simulink model "EV_TCL"  (R2020a)
settings: Solver=VariableStepAuto  StartTime=0.0  StopTime=2  RelTol=1e-3
values from neighbouring files (symbols this model uses):
  d = 0.2    [Parameters.mat]
  imax = 180    [Parameters.mat]
  Ki = 100    [Parameters.mat]
  Kp = 2.5    [Parameters.mat]
  tol = 1.0e-10    (= 1e-10)    [Prarams_TCL_test.m]
  Tsc = 5e-05    [Parameters.mat]
libraries: ee_lib x14, fl_lib x12, nesl_utility x12, sdl_lib x6, eeDiscretePi x1, eeSrmCurrentController x1
settings Model: Creator=NIKHIL  LastModifiedBy=NIKHIL

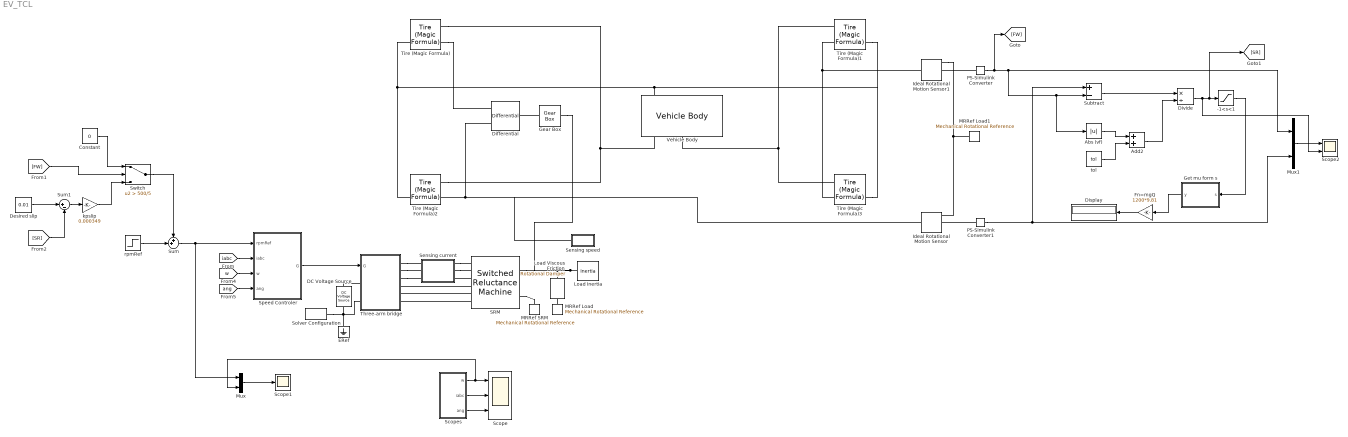
== system EV_TCL ==
  " Speed Controler " : Subsystem
  -1<s<1 : Saturate  UpperLimit=1  LowerLimit=-1
  Abs (vf) : Abs
  Add2 : Sum
  Constant : Constant  Value=0
  DC Voltage Source : fl_lib/Electrical/Electrical Sources/DC Voltage Source  v0=Vdc V
  Desired slip : Constant  Value=0.01
  Differential : sdl_lib/Gears/Differential  driveshaft_location=sdl.enum.differential_orientation.right  cd_ratio=4  friction_model=sdl.enum.gear_friction.none  mu_visc=[0, 0] N*m/(rad/s)  efficiency=[.85, .92]  temperature_TLU=[280, 300, 320] K  efficiency_ss_TLU=[.95, .9, .85]  efficiency_cd_TLU=[.95, .9, .85]  pwr_thr=[.001, .001] W  thermal_mass=50 J/K  T_init=300 K  model_inertia=simscape.enum.onoff.off  carrier_inertia=0.001 kg*m^2  planet_inertia=0.001 kg*m^2
      settings: SourceProductBaseCode=LD
  Display : Display
  Divide : Product  Inputs=*/
  ERef : fl_lib/Electrical/Electrical Elements/Electrical Reference
  Fn=mgQ : Gain  Gain=1200*9.81
  Gear Box : fl_lib/Mechanical/Mechanisms/Gear Box  ratio=5  t_in_specify=off  t_in_priority=None  t_in=0 N*m  t_in_nominal_specify=off  t_in_nominal_unit=N*m  t_in_nominal_value=1  t_out_specify=off  t_out_priority=None  t_out=0 N*m  t_out_nominal_specify=off  t_out_nominal_unit=N*m  t_out_nominal_value=1
  Get mu form s : MATLAB Function  TreatAsAtomicUnit=on
  Ideal Rotational Motion Sensor : fl_lib/Mechanical/Mechanical Sensors/Ideal Rotational Motion Sensor  wrap_angle=simscape.enum.onoff.off  offset=0 rad
  Ideal Rotational Motion Sensor1 : fl_lib/Mechanical/Mechanical Sensors/Ideal Rotational Motion Sensor  wrap_angle=simscape.enum.onoff.off  offset=0 rad
  Load Inertia : fl_lib/Mechanical/Rotational Elements/Inertia  inertia=Jm kg*m^2  w_specify=off  w_priority=High  w=0 rad/s  w_nominal_specify=off  w_nominal_unit=rad/s  w_nominal_value=1  t_specify=off  t_priority=High  t=0 N*m  t_nominal_specify=off  t_nominal_unit=N*m  t_nominal_value=1
  Load Viscous Friction : fl_lib/Mechanical/Rotational Elements/Rotational Damper  D=d N*m/(rad/s)  w_specify=off  w_priority=High  w=0 rad/s  w_nominal_specify=off  w_nominal_unit=rad/s  w_nominal_value=1  t_specify=off  t_priority=High  t=0 N*m  t_nominal_specify=off  t_nominal_unit=N*m  t_nominal_value=1
  MRRef Load : fl_lib/Mechanical/Rotational Elements/Mechanical Rotational Reference
  MRRef Load1 : fl_lib/Mechanical/Rotational Elements/Mechanical Rotational Reference
  MRRef SRM : fl_lib/Mechanical/Rotational Elements/Mechanical Rotational Reference
  Mux : Mux  Inputs=2
  Mux1 : Mux  Inputs=2
  PS-Simulink Converter : nesl_utility/PS-Simulink Converter  PhysicalDomain=network_engine_domain  SubClassName=ps_output  LeftPortType=input  RightPortType=output  PseudoPeriodic=off  Frequencies=[]  Unit=inherit  AffineConversion=off
  PS-Simulink Converter1 : nesl_utility/PS-Simulink Converter  PhysicalDomain=network_engine_domain  SubClassName=ps_output  LeftPortType=input  RightPortType=output  PseudoPeriodic=off  Frequencies=[]  Unit=inherit  AffineConversion=off
  SRM : ee_lib/Electromechanical/Reluctance & Stepper/Switched Reluctance Machine  nPoleRotor=p  Rs=Rs Ohm  stator_param=3  Rm=inf Ohm  psi_sat=0.43 Wb  Lmax=0.0046 H  Lmin=6.7e-4 H  thetaS=45 deg  thetaR=42 deg  thetaSmoothing=0.5 deg  J=0 kg*m^2  lam=0 N*m/(rad/s)  iVec=iph A  xVec=th rad  FluxMatrix=psi Wb  i_a_specify=off  i_a_priority=None  i_a=0 A  i_a_nominal_specify=off  i_a_nominal_unit=A  i_a_nominal_value=1  i_b_specify=off  i_b_priority=None  i_b=0 A  i_b_nominal_specify=off  i_b_nominal_unit=A  i_b_nominal_value=1  i_c_specify=off  i_c_priority=None  i_c=0 A  i_c_nominal_specify=off  i_c_nominal_unit=A  i_c_nominal_value=1  torque_specify=off  torque_priority=None  torque=0 N*m  torque_nominal_specify=off  torque_nominal_unit=N*m  torque_nominal_value=1  angular_velocity_specify=off  angular_velocity_priority=High  angular_velocity=0 rpm  angular_velocity_nominal_specify=off  angular_velocity_nominal_unit=rpm  angular_velocity_nominal_value=1  angular_position_diff_specify=on  angular_position_diff_priority=High  angular_position_diff=0 deg  angular_position_diff_nominal_specify=off  angular_position_diff_nominal_unit=deg  angular_position_diff_nominal_value=1  alpha=3.93e-3 1/K  Tmeas=25 degC  thermal_mass=100 J/K  rotor_thermal_mass=50 J/K  Rm_percent_rotor=50  temperatureA_specify=off  temperatureA_priority=High  temperatureA=25 degC  temperatureA_nominal_specify=off  temperatureA_nominal_unit=degC  temperatureA_nominal_value=1  temperatureB_specify=off  temperatureB_priority=High  temperatureB=25 degC  temperatureB_nominal_specify=off  temperatureB_nominal_unit=degC  temperatureB_nominal_value=1  temperatureC_specify=off  temperatureC_priority=High  temperatureC=25 degC  temperatureC_nominal_specify=off  temperatureC_nominal_unit=degC  temperatureC_nominal_value=1  temperatureR_specify=off  temperatureR_priority=High  temperatureR=25 degC  temperatureR_nominal_specify=off  temperatureR_nominal_unit=degC  temperatureR_nominal_value=1
      settings: SourceProductBaseCode=PS  InternalSimscapePortConfiguration="{\"Bottom\":[],\"Left\":[{\"id\":\"a1\",\"label\":\"a1\",\"type\":\"foundation.electrical.electrical\"},{\"id\":\"b1\",\"label\":\"b1\",\"type\":\"foundation.electrical.electrical\"},{\"id\":\"c1\",\"label\":\"c1\",\"type\":\"foundation.electrical.electrical\"},{\"id\":\"a2\",\"label\":\"a2\",\"type\":\"foundation.electrical.electrical\"},{\"id\":\"b2\",\"label\":\"b2\",\"type\":\"foundation.electrical.electrical\"},{\"id\":\"c2\",\"label\":\"c2\",\"type\":\"foundation.electrical.electrical\"}],\"Right\":[{\"id\":\"R\",\"label\":\"R\",\"type\":\"foundation.mechanical.rotational.rotational\"},{\"id\":\"C\",\"label\":\"C\",\"type\":\"foundation.mechanical.rotational.rotational\"}],\"Top\":[]}"
  Scope : Scope  NumInputPorts=3
  Scope1 : Scope
  Scope2 : Scope  NumInputPorts=2
  Scopes : Subsystem
  Sensing current : Subsystem
      mask Display: disp('iabc')
  Sensing speed : Subsystem
      mask Display: disp('w,ang')
  Solver Configuration : nesl_utility/Solver Configuration  PhysicalDomain=network_engine_domain  SubClassName=solver  LeftPortType=input  RightPortType=generic  Tones=[]  Harmonics=[]  SimulateNoise=off  Profile=off  UseLocalSampling=off  EnableSwitchedLinearOptims=on  FrequencyDomain=off  UseCCode=off  RelTol=0.001  AbsTol=1e-06  MinStep=1e-09  ToWorkspace=off  RevertToSquareIcSolve=off  NumHomotopyIterations=100  PhasorMode=off  PhasorModeNumHarmonics=1  DoDC=off  ResidualTolerance=1e-9  UseLocalSolver=on  LocalSolverChoice=NE_BACKWARD_EULER_ADVANCER  LocalSolverSampleTime=Ts  DoFixedCost=on  MaxNonlinIter=5  MaxModeIter=2  LinearAlgebra=auto  EquationFormulation=NE_TIME_EF  DelaysMemoryBudget=1024  AutomaticFiltering=on  FilteringTimeConstant=0.001  PartitionStorageMethod=AS_NEEDED  PartitionMemoryBudget=1024  PartitionMethod=FAST
  Subtract : Sum  Inputs=+-
  Sum : Sum  Inputs=++|
  Sum1 : Sum  Inputs=|+-
  Switch : Switch  Criteria=u2 > Threshold  Threshold=500/5
  Three-arm bridge : Subsystem  Tag=PublishSubsystem
  Tire (Magic Formula) : sdl_lib/Tires & Vehicles/Tire (Magic Formula)  parameterization=sdl.enum.magic_tire_model.peak  F_z1=3000 N  F_x1=3500 N  kappa1=20  B_m=10  C_m=1.9  D_m=1  E_m=0.97  fz0=4000 N  p_Cx=1.685  p_Dx=[1.21, -.037]  p_Ex=[.344, .095, -.02, 0]  p_Kx=[21.51, -.163, .245]  p_Hx=[-.002, .002]  p_Vx=[0, 0]  v_tr_thr=0.1 m/s  r_e=0.3 m  model_compliance=0  stiffness=1e6 N/m  damping=1000 N/(m/s)  model_inertia=0  inertia=1 kg*m^2  initial_velocity=0 rad/s  model_resistance=0  resistance_model=1  coeff=0.015  p_tire=250e3 Pa  alpha=-0.003  beta=0.97  coeff_a=84e-4  coeff_b=6.2e-4 s/m  coeff_c=1.6e-4 s^2/m^2  v_thr=0.001 m/s
  Tire (Magic Formula)1 : sdl_lib/Tires & Vehicles/Tire (Magic Formula)  parameterization=sdl.enum.magic_tire_model.peak  F_z1=3000 N  F_x1=3500 N  kappa1=10  B_m=10  C_m=1.9  D_m=1  E_m=0.97  fz0=4000 N  p_Cx=1.685  p_Dx=[1.21, -.037]  p_Ex=[.344, .095, -.02, 0]  p_Kx=[21.51, -.163, .245]  p_Hx=[-.002, .002]  p_Vx=[0, 0]  v_tr_thr=0.1 m/s  r_e=0.3 m  model_compliance=0  stiffness=1e6 N/m  damping=1000 N/(m/s)  model_inertia=0  inertia=1 kg*m^2  initial_velocity=0 rad/s  model_resistance=0  resistance_model=1  coeff=0.015  p_tire=250e3 Pa  alpha=-0.003  beta=0.97  coeff_a=84e-4  coeff_b=6.2e-4 s/m  coeff_c=1.6e-4 s^2/m^2  v_thr=0.001 m/s
  Tire (Magic Formula)2 : sdl_lib/Tires & Vehicles/Tire (Magic Formula)  parameterization=sdl.enum.magic_tire_model.peak  F_z1=3000 N  F_x1=3500 N  kappa1=20  B_m=10  C_m=1.9  D_m=1  E_m=0.97  fz0=4000 N  p_Cx=1.685  p_Dx=[1.21, -.037]  p_Ex=[.344, .095, -.02, 0]  p_Kx=[21.51, -.163, .245]  p_Hx=[-.002, .002]  p_Vx=[0, 0]  v_tr_thr=0.1 m/s  r_e=0.3 m  model_compliance=0  stiffness=1e6 N/m  damping=1000 N/(m/s)  model_inertia=0  inertia=1 kg*m^2  initial_velocity=0 rad/s  model_resistance=0  resistance_model=1  coeff=0.015  p_tire=250e3 Pa  alpha=-0.003  beta=0.97  coeff_a=84e-4  coeff_b=6.2e-4 s/m  coeff_c=1.6e-4 s^2/m^2  v_thr=0.001 m/s
  Tire (Magic Formula)3 : sdl_lib/Tires & Vehicles/Tire (Magic Formula)  parameterization=sdl.enum.magic_tire_model.peak  F_z1=3000 N  F_x1=3500 N  kappa1=10  B_m=10  C_m=1.9  D_m=1  E_m=0.97  fz0=4000 N  p_Cx=1.685  p_Dx=[1.21, -.037]  p_Ex=[.344, .095, -.02, 0]  p_Kx=[21.51, -.163, .245]  p_Hx=[-.002, .002]  p_Vx=[0, 0]  v_tr_thr=0.1 m/s  r_e=0.3 m  model_compliance=0  stiffness=1e6 N/m  damping=1000 N/(m/s)  model_inertia=0  inertia=1 kg*m^2  initial_velocity=0 rad/s  model_resistance=0  resistance_model=1  coeff=0.015  p_tire=250e3 Pa  alpha=-0.003  beta=0.97  coeff_a=84e-4  coeff_b=6.2e-4 s/m  coeff_c=1.6e-4 s^2/m^2  v_thr=0.001 m/s
  Vehicle Body : sdl_lib/Tires & Vehicles/Vehicle Body  mass=1200 kg  n_w=2  x_f=1.4 m  x_r=1.6 m  y_c=0.5 m  mass_var=simscape.enum.onoff.off  model_pitch=simscape.enum.onoff.off  inertia=4000 kg*m^2  suspension_model=sdl.enum.linearTLU.linear  k_f=1e4 N/m  b_f=1e4 N/(m/s)  k_r=1e4 N/m  b_r=1e4 N/(m/s)  k_f_TLU=[-2000, -1000, 0, 1000, 2000] N  x_f_TLU=[-.4, -.2, 0, .2, .4] m  b_f_TLU=[-200, -100, 0, 100, 200] N  v_f_TLU=[-4, -2, 0, 2, 4] m/s  k_r_TLU=[-2000, -1000, 0, 1000, 2000] N  x_r_TLU=[-.4, -.2, 0, .2, .4] m  b_r_TLU=[-200, -100, 0, 100, 200] N  v_r_TLU=[-4, -2, 0, 2, 4] m/s  interp_method=simscape.enum.interpolation.linear  extrap_method=simscape.enum.extrapolation.linear  model_hardstop=simscape.enum.onoff.off  upper_bound_f=.25 m  lower_bound_f=-.25 m  stop_k_f=1e6 N/m  stop_b_f=150 N/(m/s)  upper_bound_r=.25 m  lower_bound_r=-.25 m  stop_k_r=1e6 N/m  stop_b_r=150 N/(m/s)  initial_pitch=0 rad  initial_pitch_rate=0 rad/s  g=9.81 m/s^2  liftoff_warning=simscape.enum.onoff.off  area=3 m^2  Cd=0.4  rho=1.18 kg/m^3  v_specify=off  v_priority=High  v=0 m/s  v_nominal_specify=off  v_nominal_unit=m/s  v_nominal_value=1
  kpslip : Gain  Gain=0.000349
  rpmRef : Step  Time=0.5  After=500  SampleTime=0
  tol : Constant  Value=tol
  wires:
  Mux/1 -> Scope1/1
  [iabc] -> " Speed Controler "/2(iabc)
  Scopes/2(iabc) -> Scope/2
  Scopes/3(ang) -> Scope/3
  Scopes/1(w) -> Mux/2, Scope/1
  " Speed Controler "/1(G) -> Three-arm bridge/1(G)
  [w] -> " Speed Controler "/3(w)
  [ang] -> " Speed Controler "/4(ang)
  Mux1/1 -> Scope2/1
  -1<s<1/1 -> Get mu form s/1(s)
  tol/1 -> Add2/2
  Divide/1 -> Scope2/2, [SR], -1<s<1/1
  Add2/1 -> Divide/2
  Get mu form s/1(y) -> Fn=mgQ/1
  Fn=mgQ/1 -> Display/1
  Abs (vf)/1 -> Add2/1
  Subtract/1 -> Divide/1
  PS-Simulink Converter1/1 -> Mux1/2, Subtract/1
  PS-Simulink Converter/1 -> [FW], Abs (vf)/1, Subtract/2, Mux1/1
  Constant/1 -> Switch/1
  Sum1/1 -> kpslip/1
  Desired slip/1 -> Sum1/1
  kpslip/1 -> Switch/3
  [FW] -> Switch/2
  [SR] -> Sum1/2
  rpmRef/1 -> Sum/2
  Sum/1 -> Mux/1, " Speed Controler "/1(rpmRef)
  Switch/1 -> Sum/1
  connections:
  Differential/RConn2 -- Sensing speed/LConn1 -- Ideal Rotational Motion Sensor/LConn1 -- Tire (Magic Formula)2/LConn2
  Tire (Magic Formula)/LConn2 -- Differential/RConn1
  Gear Box/LConn1 -- Differential/LConn1
  Vehicle Body/LConn1 -- Tire (Magic Formula)1/RConn2 -- Tire (Magic Formula)3/RConn2 -- Tire (Magic Formula)2/RConn2 -- Tire (Magic Formula)/RConn2
  Tire (Magic Formula)/LConn1 -- Tire (Magic Formula)2/LConn1 -- Vehicle Body/RConn1
  Tire (Magic Formula)1/LConn1 -- Tire (Magic Formula)3/LConn1 -- Vehicle Body/RConn2
  Tire (Magic Formula)3/LConn2 -- Ideal Rotational Motion Sensor1/LConn1 -- Tire (Magic Formula)1/LConn2
  Solver Configuration/RConn1 -- ERef/LConn1 -- DC Voltage Source/RConn1 -- Three-arm bridge/LConn2
  Load Inertia/LConn1 -- Gear Box/RConn1 -- SRM/RConn1 -- Load Viscous Friction/LConn1
  SRM/LConn5 -- Three-arm bridge/RConn5
  Sensing current/RConn1 -- SRM/LConn1
  SRM/LConn4 -- Three-arm bridge/RConn4
  Three-arm bridge/LConn1 -- DC Voltage Source/LConn1
  SRM/LConn6 -- Three-arm bridge/RConn6
  SRM/RConn2 -- MRRef SRM/LConn1
  Three-arm bridge/RConn3 -- Sensing current/LConn3
  Three-arm bridge/RConn2 -- Sensing current/LConn2
  Three-arm bridge/RConn1 -- Sensing current/LConn1
  SRM/LConn3 -- Sensing current/RConn3
  MRRef Load/LConn1 -- Load Viscous Friction/RConn1
  Sensing current/RConn2 -- SRM/LConn2
  PS-Simulink Converter/LConn1 -- Ideal Rotational Motion Sensor1/RConn2
  PS-Simulink Converter1/LConn1 -- Ideal Rotational Motion Sensor/RConn2
  Ideal Rotational Motion Sensor1/RConn1 -- MRRef Load1/LConn1 -- Ideal Rotational Motion Sensor/RConn1

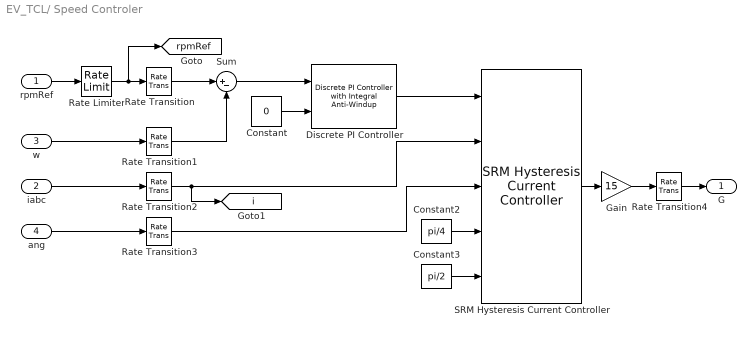
== system EV_TCL/ Speed Controler  ==
  rpmRef : Inport
  iabc : Inport  Port=2
  w : Inport  Port=3
  ang : Inport  Port=4
  Constant : Constant  Value=0  SampleTime=Tsc
  Constant2 : Constant  Value=pi/4  SampleTime=Tsc
  Constant3 : Constant  Value=pi/2  SampleTime=Tsc
  Discrete PI Controller : eeDiscretePi/Discrete PI Controller with Integral Anti-Windup  Kp=Kp  Ki=Ki  x0=0  B=imax  A=0  Ts=Tsc
      settings: SourceProductBaseCode=PS
  Gain : Gain  Gain=15
  Rate Limiter : RateLimiter  RisingSlewLimit=2000  FallingSlewLimit=-2000  SampleTimeMode=inherited
      settings: AttributesFormatString=2000 rpm/s
  Rate Transition{,1..3} (4 alike) : RateTransition  OutPortSampleTime=Tsc
  Rate Transition4 : RateTransition
  SRM Hysteresis Current Controller : eeSrmCurrentController/SRM Hysteresis Current Controller  beta=pi/2  h=10  Ts=Tsc
      settings: SourceProductBaseCode=PS
  Sum : Sum  Inputs=|+-
  G : Outport  VectorParamsAs1DForOutWhenUnconnected=off
  tag scope: i=global, rpmRef=global
  wires:
  Rate Transition4/1 -> G/1
  w/1 -> Rate Transition1/1
  rpmRef/1 -> Rate Limiter/1
  Sum/1 -> Discrete PI Controller/1
  SRM Hysteresis Current Controller/1 -> Gain/1
  iabc/1 -> Rate Transition2/1
  ang/1 -> Rate Transition3/1
  Rate Transition/1 -> Sum/1
  Rate Transition1/1 -> Sum/2
  Rate Transition2/1 -> [i], SRM Hysteresis Current Controller/2
  Rate Limiter/1 -> [rpmRef], Rate Transition/1
  Constant/1 -> Discrete PI Controller/2
  Discrete PI Controller/1 -> SRM Hysteresis Current Controller/1
  Rate Transition3/1 -> SRM Hysteresis Current Controller/3
  Constant2/1 -> SRM Hysteresis Current Controller/4
  Constant3/1 -> SRM Hysteresis Current Controller/5
  Gain/1 -> Rate Transition4/1

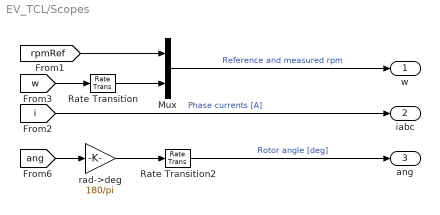
== system EV_TCL/Scopes ==
  Mux : Mux  Inputs=2
  Rate Transition : RateTransition  OutPortSampleTime=Ts
  Rate Transition2 : RateTransition  OutPortSampleTime=Ts
  rad->deg : Gain  Gain=180/pi
  w : Outport  VectorParamsAs1DForOutWhenUnconnected=off
  iabc : Outport  Port=2  VectorParamsAs1DForOutWhenUnconnected=off
  ang : Outport  Port=3  VectorParamsAs1DForOutWhenUnconnected=off
  wires:
  [w] -> Rate Transition/1
  [i] -> iabc/1  "Phase currents [A]"
  [rpmRef] -> Mux/1
  rad->deg/1 -> Rate Transition2/1
  Rate Transition/1 -> Mux/2
  Rate Transition2/1 -> ang/1  "Rotor angle [deg]"
  [ang] -> rad->deg/1
  Mux/1 -> w/1  "Reference and measured rpm"

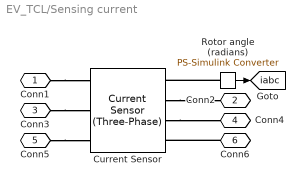
== system EV_TCL/Sensing current ==
  Current Sensor : ee_lib/Sensors & Transducers/Current Sensor (Three-Phase)
      settings: InternalSimscapePortConfiguration="{\"Bottom\":[],\"Left\":[{\"id\":\"a1\",\"label\":\"a1\",\"type\":\"foundation.electrical.electrical\"},{\"id\":\"b1\",\"label\":\"b1\",\"type\":\"foundation.electrical.electrical\"},{\"id\":\"c1\",\"label\":\"c1\",\"type\":\"foundation.electrical.electrical\"}],\"Right\":[{\"id\":\"I_output\",\"label\":\"I\",\"type\":\"output\"},{\"id\":\"a2\",\"label\":\"a2\",\"type\":\"foundation.electrical.electrical\"},{\"id\":\"b2\",\"label\":\"b2\",\"type\":\"foundation.electrical.electrical\"},{\"id\":\"c2\",\"label\":\"c2\",\"type\":\"foundation.electrical.electrical\"}],\"Top\":[]}"
  Rotor angle (radians) : nesl_utility/PS-Simulink Converter  PhysicalDomain=network_engine_domain  SubClassName=ps_output  LeftPortType=input  RightPortType=output  PseudoPeriodic=off  Frequencies=[]  Unit=A  AffineConversion=off
  Conn1 : PMIOPort  Side=Left
  Conn2 : PMIOPort  Port=2  Side=Right
  Conn3 : PMIOPort  Port=3  Side=Left
  Conn4 : PMIOPort  Port=4  Side=Right
  Conn5 : PMIOPort  Port=5  Side=Left
  Conn6 : PMIOPort  Port=6  Side=Right
  tag scope: iabc=global
  wires:
  Rotor angle (radians)/1 -> [iabc]
  connections:
  Rotor angle (radians)/LConn1 -- Current Sensor/RConn1
  Conn1/RConn1 -- Current Sensor/LConn1
  Current Sensor/RConn2 -- Conn2/RConn1
  Conn3/RConn1 -- Current Sensor/LConn2
  Conn5/RConn1 -- Current Sensor/LConn3
  Conn6/RConn1 -- Current Sensor/RConn4
  Current Sensor/RConn3 -- Conn4/RConn1

== system EV_TCL/Sensing speed ==
  Speed sensing : Subsystem
  Conn1 : PMIOPort  Side=Left
  tag scope: ang=global, w=global
  wires:
  Speed sensing/2(rpm) -> [w]
  Speed sensing/1(Angle) -> [ang]
  connections:
  Conn1/RConn1 -- Speed sensing/LConn1

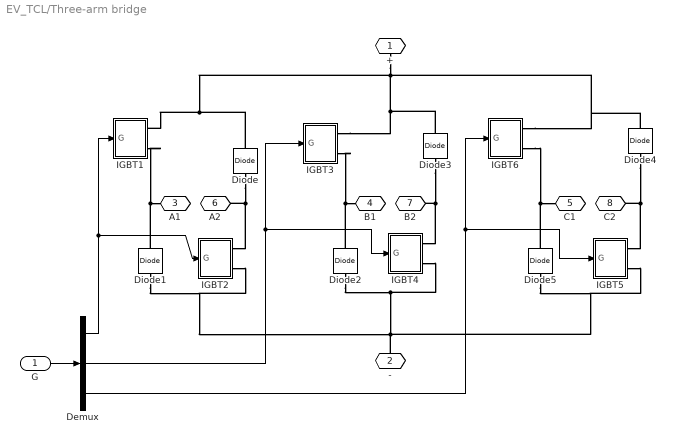
== system EV_TCL/Three-arm bridge ==
  G : Inport
  Demux : Demux  Outputs=3
  Diode{,1..5} (6 alike) : ee_lib/Semiconductors & Converters/Diode  ModelType=ee.enum.diode.modelType.pwl  Vf=0.6 V  Ron=0.3 Ohm  Goff=1e-8 1/Ohm  prmExp=ee.enum.diode.expParam.useTwo  I12=[.0137, .545] A  V12=[.6, .7] V  IS=1e-12 A  ec=1  I1=0.0137 A  V1=0.6 V  RS=0 Ohm  Tmeas=25 degC  N_series=1  N_parallel=1  Rz=0.3 Ohm  BV=inf V  C_param=ee.enum.diode.capParam.fixed  CJ=0 pF  CJ0=5 pF  VJ=1 V  Mgrad=0.5  Vvec=[.1, 10, 100] V  Cvec=[3.5, 1, .4] pF  FC=0.5  Q_param=ee.enum.diode.recoveryParam.off  iRM=-7.15 A  iF=4 A  didt=-750 A/us  trr_factor=3  trr=115 ns  Qrr=1500 s*uA  TT=50 ns  tau=100 ns  T_param=ee.enum.diode.temperatureParam.off  IS_T2=1.25e-7 A  I1_T2=0.245 A  V1_T2=0.5 V  Tmeas2=125 degC  EG_param=ee.enum.diode.egapParam.material_si  EG=1.11 eV  XTI_param=ee.enum.diode.xtiParam.pn  XTI=3  dBVdT=0 V/K  Tdevice=25 degC  i_specify=off  i_priority=None  i=0 A  i_nominal_specify=off  i_nominal_unit=A  i_nominal_value=1  v_specify=off  v_priority=None  v=0 V  v_nominal_specify=off  v_nominal_unit=V  v_nominal_value=1  i_capacitor_specify=off  i_capacitor_priority=None  i_capacitor=0 A  i_capacitor_nominal_specify=off  i_capacitor_nominal_unit=A  i_capacitor_nominal_value=1  v_capacitor_specify=off  v_capacitor_priority=None  v_capacitor=0 V  v_capacitor_nominal_specify=off  v_capacitor_nominal_unit=V  v_capacitor_nominal_value=1  power_dissipated_specify=off  power_dissipated_priority=None  power_dissipated=0 W  power_dissipated_nominal_specify=off  power_dissipated_nominal_unit=W  power_dissipated_nominal_value=1  thermal_network_parameterization=ee.enum.thermalNetworkTopology.cauer  Rth=[0, 10] K/W  Rth_Foster=[4, 6] K/W  thermal_mass_parameterization=ee.enum.thermalNetwork.timeconstant  thermal_mass=[0, 1] J/K  thermal_mass_Foster=[1.5, 3] J/K  thermal_time_constant=[0, 10] s  thermal_time_constant_Foster=[6, 18] s  thermal_mass_initial_temperatures=[25, 25] degC
  IGBT1 : Subsystem
  IGBT2 : Subsystem
  IGBT3 : Subsystem
  IGBT4 : Subsystem
  IGBT5 : Subsystem
  IGBT6 : Subsystem
  + : PMIOPort  Side=Left
  - : PMIOPort  Port=2  Side=Left
  A1 : PMIOPort  Port=3  Side=Right
  B1 : PMIOPort  Port=4  Side=Right
  C1 : PMIOPort  Port=5  Side=Right
  A2 : PMIOPort  Port=6  Side=Right
  B2 : PMIOPort  Port=7  Side=Right
  C2 : PMIOPort  Port=8  Side=Right
  wires:
  Demux/1 -> IGBT1/1(G), IGBT2/1(G)
  Demux/2 -> IGBT3/1(G), IGBT4/1(G)
  Demux/3 -> IGBT6/1(G), IGBT5/1(G)
  G/1 -> Demux/1
  connections:
  IGBT1/RConn2 -- A1/RConn1 -- Diode1/RConn1
  Diode2/LConn1 -- -/RConn1 -- IGBT2/RConn2 -- Diode1/LConn1 -- IGBT5/RConn2 -- Diode5/LConn1 -- IGBT4/RConn2
  Diode3/RConn1 -- IGBT6/RConn1 -- Diode4/RConn1 -- Diode/RConn1 -- IGBT1/RConn1 -- +/RConn1 -- IGBT3/RConn1
  Diode5/RConn1 -- C1/RConn1 -- IGBT6/RConn2
  Diode2/RConn1 -- B1/RConn1 -- IGBT3/RConn2
  Diode/LConn1 -- A2/RConn1 -- IGBT2/RConn1
  Diode3/LConn1 -- B2/RConn1 -- IGBT4/RConn1
  Diode4/LConn1 -- C2/RConn1 -- IGBT5/RConn1

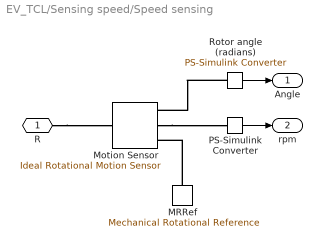
== system EV_TCL/Sensing speed/Speed sensing ==
  MRRef : fl_lib/Mechanical/Rotational Elements/Mechanical Rotational Reference
  Motion Sensor : fl_lib/Mechanical/Mechanical Sensors/Ideal Rotational Motion Sensor  wrap_angle=simscape.enum.onoff.off  offset=0 deg
  PS-Simulink Converter : nesl_utility/PS-Simulink Converter  PhysicalDomain=network_engine_domain  SubClassName=ps_output  LeftPortType=input  RightPortType=output  PseudoPeriodic=off  Frequencies=[]  Unit=rpm  AffineConversion=off
  Rotor angle (radians) : nesl_utility/PS-Simulink Converter  PhysicalDomain=network_engine_domain  SubClassName=ps_output  LeftPortType=input  RightPortType=output  PseudoPeriodic=off  Frequencies=[]  Unit=rad  AffineConversion=off
  R : PMIOPort  Side=Left
  Angle : Outport  VectorParamsAs1DForOutWhenUnconnected=off
  rpm : Outport  Port=2  VectorParamsAs1DForOutWhenUnconnected=off
  wires:
  PS-Simulink Converter/1 -> rpm/1
  Rotor angle (radians)/1 -> Angle/1
  connections:
  R/RConn1 -- Motion Sensor/LConn1
  Rotor angle (radians)/LConn1 -- Motion Sensor/RConn3
  Motion Sensor/RConn2 -- PS-Simulink Converter/LConn1
  MRRef/LConn1 -- Motion Sensor/RConn1

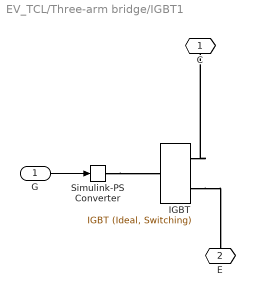
== system EV_TCL/Three-arm bridge/IGBT1 ==
  G : Inport
  IGBT : ee_lib/Semiconductors & Converters/IGBT (Ideal, Switching)  Vf=6 V  Ron=0.01 Ohm  Goff=1e-5 1/Ohm  Vth=6 V  diode_param=2  diode_Vf=0.6 V  diode_Ron=0.03 Ohm  diode_Goff=1e-5 1/Ohm  diode_C=5e-8 F  diode_iRM=-235 A  diode_iF=300 A  diode_idot=-50 A/us  diode_trr_param=1  diode_trr_factor=3  diode_trr=15 us  diode_Qrr=1.5e+3 s*uA  thermal_loss_option=2  Voff=300 V  Tau=1e-4 s  Tj=[298.15, 398.15] K  Iout_scalar=600 A  Eon_scalar=22.86e-3 J  Eoff_scalar=17.14e-3 J  Von_scalar=2.7 V  Iout_data=[0, 10, 50, 100, 200, 400, 600] A  Eon_data=[0, .29, 1.43, 2.86, 5.71, 13.14, 22.86; 0, .57, 2.63, 5.14, 10.29, 20.57, 30.29] * 1e-3 J  Eoff_data=[0, .21, 1.07, 2.14, 4.29, 9.86, 17.14; 0, .43, 1.97, 3.86, 7.71, 15.43, 22.71] * 1e-3 J  Von_data=[0, 1.1, 1.3, 1.45, 1.75, 2.25, 2.7; 0, 1, 1.15, 1.35, 1.7, 2.35, 3] V
  Simulink-PS Converter : nesl_utility/Simulink-PS Converter  PhysicalDomain=network_engine_domain  SubClassName=ps_input  LeftPortType=input  RightPortType=output  PseudoPeriodic=off  Frequencies=[]  NoiseDistribution=none  NoiseParameters=[]  Unit=V  AffineConversion=off  FilteringAndDerivatives=zero  SimscapeFilterOrder=1  InputFilterTimeConstant=.001  UdotUserProvided=1
  C : PMIOPort  Side=Right
  E : PMIOPort  Port=2  Side=Right
  wires:
  G/1 -> Simulink-PS Converter/1
  connections:
  IGBT/RConn1 -- C/RConn1
  IGBT/RConn2 -- E/RConn1
  Simulink-PS Converter/RConn1 -- IGBT/LConn1

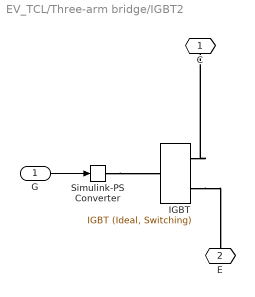
== system EV_TCL/Three-arm bridge/IGBT2 ==
  G : Inport
  IGBT : ee_lib/Semiconductors & Converters/IGBT (Ideal, Switching)  Vf=6 V  Ron=0.01 Ohm  Goff=1e-5 1/Ohm  Vth=6 V  diode_param=2  diode_Vf=0.6 V  diode_Ron=0.03 Ohm  diode_Goff=1e-5 1/Ohm  diode_C=5e-8 F  diode_iRM=-235 A  diode_iF=300 A  diode_idot=-50 A/us  diode_trr_param=1  diode_trr_factor=3  diode_trr=15 us  diode_Qrr=1.5e+3 s*uA  thermal_loss_option=2  Voff=300 V  Tau=1e-4 s  Tj=[298.15, 398.15] K  Iout_scalar=600 A  Eon_scalar=22.86e-3 J  Eoff_scalar=17.14e-3 J  Von_scalar=2.7 V  Iout_data=[0, 10, 50, 100, 200, 400, 600] A  Eon_data=[0, .29, 1.43, 2.86, 5.71, 13.14, 22.86; 0, .57, 2.63, 5.14, 10.29, 20.57, 30.29] * 1e-3 J  Eoff_data=[0, .21, 1.07, 2.14, 4.29, 9.86, 17.14; 0, .43, 1.97, 3.86, 7.71, 15.43, 22.71] * 1e-3 J  Von_data=[0, 1.1, 1.3, 1.45, 1.75, 2.25, 2.7; 0, 1, 1.15, 1.35, 1.7, 2.35, 3] V
  Simulink-PS Converter : nesl_utility/Simulink-PS Converter  PhysicalDomain=network_engine_domain  SubClassName=ps_input  LeftPortType=input  RightPortType=output  PseudoPeriodic=off  Frequencies=[]  NoiseDistribution=none  NoiseParameters=[]  Unit=V  AffineConversion=off  FilteringAndDerivatives=zero  SimscapeFilterOrder=1  InputFilterTimeConstant=.001  UdotUserProvided=1
  C : PMIOPort  Side=Right
  E : PMIOPort  Port=2  Side=Right
  wires:
  G/1 -> Simulink-PS Converter/1
  connections:
  Simulink-PS Converter/RConn1 -- IGBT/LConn1
  IGBT/RConn2 -- E/RConn1
  IGBT/RConn1 -- C/RConn1

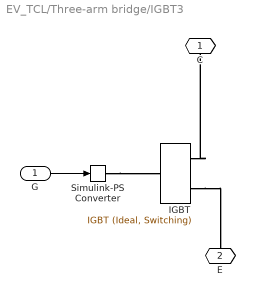
== system EV_TCL/Three-arm bridge/IGBT3 ==
  G : Inport
  IGBT : ee_lib/Semiconductors & Converters/IGBT (Ideal, Switching)  Vf=6 V  Ron=0.01 Ohm  Goff=1e-5 1/Ohm  Vth=6 V  diode_param=2  diode_Vf=0.6 V  diode_Ron=0.03 Ohm  diode_Goff=1e-5 1/Ohm  diode_C=5e-8 F  diode_iRM=-235 A  diode_iF=300 A  diode_idot=-50 A/us  diode_trr_param=1  diode_trr_factor=3  diode_trr=15 us  diode_Qrr=1.5e+3 s*uA  thermal_loss_option=2  Voff=300 V  Tau=1e-4 s  Tj=[298.15, 398.15] K  Iout_scalar=600 A  Eon_scalar=22.86e-3 J  Eoff_scalar=17.14e-3 J  Von_scalar=2.7 V  Iout_data=[0, 10, 50, 100, 200, 400, 600] A  Eon_data=[0, .29, 1.43, 2.86, 5.71, 13.14, 22.86; 0, .57, 2.63, 5.14, 10.29, 20.57, 30.29] * 1e-3 J  Eoff_data=[0, .21, 1.07, 2.14, 4.29, 9.86, 17.14; 0, .43, 1.97, 3.86, 7.71, 15.43, 22.71] * 1e-3 J  Von_data=[0, 1.1, 1.3, 1.45, 1.75, 2.25, 2.7; 0, 1, 1.15, 1.35, 1.7, 2.35, 3] V
  Simulink-PS Converter : nesl_utility/Simulink-PS Converter  PhysicalDomain=network_engine_domain  SubClassName=ps_input  LeftPortType=input  RightPortType=output  PseudoPeriodic=off  Frequencies=[]  NoiseDistribution=none  NoiseParameters=[]  Unit=V  AffineConversion=off  FilteringAndDerivatives=zero  SimscapeFilterOrder=1  InputFilterTimeConstant=.001  UdotUserProvided=1
  C : PMIOPort  Side=Right
  E : PMIOPort  Port=2  Side=Right
  wires:
  G/1 -> Simulink-PS Converter/1
  connections:
  IGBT/RConn1 -- C/RConn1
  IGBT/RConn2 -- E/RConn1
  Simulink-PS Converter/RConn1 -- IGBT/LConn1

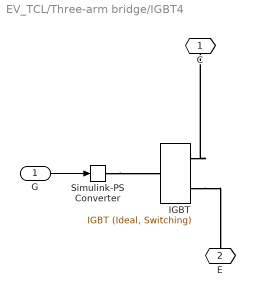
== system EV_TCL/Three-arm bridge/IGBT4 ==
  G : Inport
  IGBT : ee_lib/Semiconductors & Converters/IGBT (Ideal, Switching)  Vf=6 V  Ron=0.01 Ohm  Goff=1e-5 1/Ohm  Vth=6 V  diode_param=2  diode_Vf=0.6 V  diode_Ron=0.03 Ohm  diode_Goff=1e-5 1/Ohm  diode_C=5e-8 F  diode_iRM=-235 A  diode_iF=300 A  diode_idot=-50 A/us  diode_trr_param=1  diode_trr_factor=3  diode_trr=15 us  diode_Qrr=1.5e+3 s*uA  thermal_loss_option=2  Voff=300 V  Tau=1e-4 s  Tj=[298.15, 398.15] K  Iout_scalar=600 A  Eon_scalar=22.86e-3 J  Eoff_scalar=17.14e-3 J  Von_scalar=2.7 V  Iout_data=[0, 10, 50, 100, 200, 400, 600] A  Eon_data=[0, .29, 1.43, 2.86, 5.71, 13.14, 22.86; 0, .57, 2.63, 5.14, 10.29, 20.57, 30.29] * 1e-3 J  Eoff_data=[0, .21, 1.07, 2.14, 4.29, 9.86, 17.14; 0, .43, 1.97, 3.86, 7.71, 15.43, 22.71] * 1e-3 J  Von_data=[0, 1.1, 1.3, 1.45, 1.75, 2.25, 2.7; 0, 1, 1.15, 1.35, 1.7, 2.35, 3] V
  Simulink-PS Converter : nesl_utility/Simulink-PS Converter  PhysicalDomain=network_engine_domain  SubClassName=ps_input  LeftPortType=input  RightPortType=output  PseudoPeriodic=off  Frequencies=[]  NoiseDistribution=none  NoiseParameters=[]  Unit=V  AffineConversion=off  FilteringAndDerivatives=zero  SimscapeFilterOrder=1  InputFilterTimeConstant=.001  UdotUserProvided=1
  C : PMIOPort  Side=Right
  E : PMIOPort  Port=2  Side=Right
  wires:
  G/1 -> Simulink-PS Converter/1
  connections:
  Simulink-PS Converter/RConn1 -- IGBT/LConn1
  IGBT/RConn2 -- E/RConn1
  IGBT/RConn1 -- C/RConn1

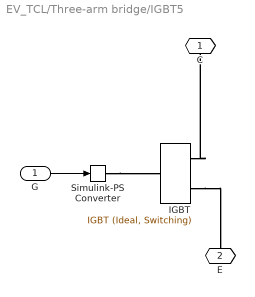
== system EV_TCL/Three-arm bridge/IGBT5 ==
  G : Inport
  IGBT : ee_lib/Semiconductors & Converters/IGBT (Ideal, Switching)  Vf=6 V  Ron=0.01 Ohm  Goff=1e-5 1/Ohm  Vth=6 V  diode_param=2  diode_Vf=0.6 V  diode_Ron=0.03 Ohm  diode_Goff=1e-5 1/Ohm  diode_C=5e-8 F  diode_iRM=-235 A  diode_iF=300 A  diode_idot=-50 A/us  diode_trr_param=1  diode_trr_factor=3  diode_trr=15 us  diode_Qrr=1.5e+3 s*uA  thermal_loss_option=2  Voff=300 V  Tau=1e-4 s  Tj=[298.15, 398.15] K  Iout_scalar=600 A  Eon_scalar=22.86e-3 J  Eoff_scalar=17.14e-3 J  Von_scalar=2.7 V  Iout_data=[0, 10, 50, 100, 200, 400, 600] A  Eon_data=[0, .29, 1.43, 2.86, 5.71, 13.14, 22.86; 0, .57, 2.63, 5.14, 10.29, 20.57, 30.29] * 1e-3 J  Eoff_data=[0, .21, 1.07, 2.14, 4.29, 9.86, 17.14; 0, .43, 1.97, 3.86, 7.71, 15.43, 22.71] * 1e-3 J  Von_data=[0, 1.1, 1.3, 1.45, 1.75, 2.25, 2.7; 0, 1, 1.15, 1.35, 1.7, 2.35, 3] V
  Simulink-PS Converter : nesl_utility/Simulink-PS Converter  PhysicalDomain=network_engine_domain  SubClassName=ps_input  LeftPortType=input  RightPortType=output  PseudoPeriodic=off  Frequencies=[]  NoiseDistribution=none  NoiseParameters=[]  Unit=V  AffineConversion=off  FilteringAndDerivatives=zero  SimscapeFilterOrder=1  InputFilterTimeConstant=.001  UdotUserProvided=1
  C : PMIOPort  Side=Right
  E : PMIOPort  Port=2  Side=Right
  wires:
  G/1 -> Simulink-PS Converter/1
  connections:
  IGBT/RConn1 -- C/RConn1
  IGBT/RConn2 -- E/RConn1
  Simulink-PS Converter/RConn1 -- IGBT/LConn1

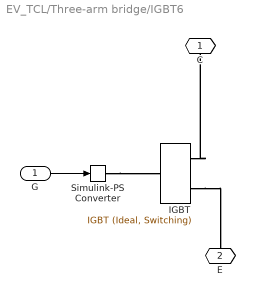
== system EV_TCL/Three-arm bridge/IGBT6 ==
  G : Inport
  IGBT : ee_lib/Semiconductors & Converters/IGBT (Ideal, Switching)  Vf=6 V  Ron=0.01 Ohm  Goff=1e-5 1/Ohm  Vth=6 V  diode_param=2  diode_Vf=0.6 V  diode_Ron=0.03 Ohm  diode_Goff=1e-5 1/Ohm  diode_C=5e-8 F  diode_iRM=-235 A  diode_iF=300 A  diode_idot=-50 A/us  diode_trr_param=1  diode_trr_factor=3  diode_trr=15 us  diode_Qrr=1.5e+3 s*uA  thermal_loss_option=2  Voff=300 V  Tau=1e-4 s  Tj=[298.15, 398.15] K  Iout_scalar=600 A  Eon_scalar=22.86e-3 J  Eoff_scalar=17.14e-3 J  Von_scalar=2.7 V  Iout_data=[0, 10, 50, 100, 200, 400, 600] A  Eon_data=[0, .29, 1.43, 2.86, 5.71, 13.14, 22.86; 0, .57, 2.63, 5.14, 10.29, 20.57, 30.29] * 1e-3 J  Eoff_data=[0, .21, 1.07, 2.14, 4.29, 9.86, 17.14; 0, .43, 1.97, 3.86, 7.71, 15.43, 22.71] * 1e-3 J  Von_data=[0, 1.1, 1.3, 1.45, 1.75, 2.25, 2.7; 0, 1, 1.15, 1.35, 1.7, 2.35, 3] V
  Simulink-PS Converter : nesl_utility/Simulink-PS Converter  PhysicalDomain=network_engine_domain  SubClassName=ps_input  LeftPortType=input  RightPortType=output  PseudoPeriodic=off  Frequencies=[]  NoiseDistribution=none  NoiseParameters=[]  Unit=V  AffineConversion=off  FilteringAndDerivatives=zero  SimscapeFilterOrder=1  InputFilterTimeConstant=.001  UdotUserProvided=1
  C : PMIOPort  Side=Right
  E : PMIOPort  Port=2  Side=Right
  wires:
  G/1 -> Simulink-PS Converter/1
  connections:
  Simulink-PS Converter/RConn1 -- IGBT/LConn1
  IGBT/RConn2 -- E/RConn1
  IGBT/RConn1 -- C/RConn1

== matlab function EV_TCL/Get mu form s ==
  data: s input; y output
function y = fcn(s)
%#codegen

%slip is already saturated
%ONLY DEFINED from 1 tp\o -1
a1=1.63;
a2=-0.9;
a3=-0.1;

c1=-27;
c2=-15;

if s<0
    s=abs(s);
    mu=-(a1*(1-exp(c1*s))+a2*(1-exp(c2*s))+a3*s);
else
    mu=a1*(1-exp(c1*s))+a2*(1-exp(c2*s))+a3*s;
end

y = mu;
